simulink model "torque_catalogue"  (R2023b)
settings: Solver=VariableStepAuto  StartTime=0.0  StopTime=10.0  RelTol=1e-3
values from neighbouring files (symbols this model uses):
  ni = 13    [ParameterizeMotorTorqueData.mat]
  nx = 46    [ParameterizeMotorTorqueData.mat]
libraries: fl_lib x20, nesl_utility x9, ee_lib x3
settings Model: Creator=simon  LastModifiedBy=simon
settings SimscapeCC: SimscapeLogType=all  SimscapeLogSimulationStatistics=on

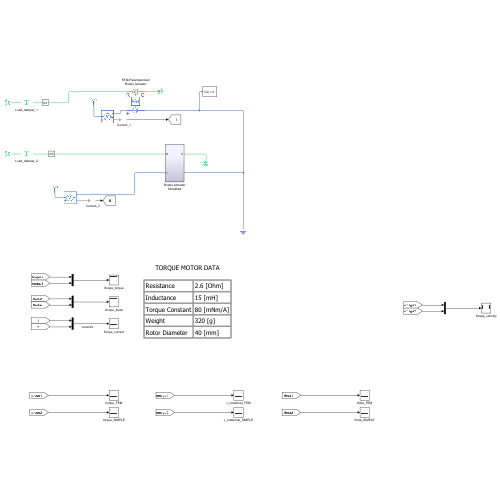
[thumbnail: Simulink's stored preview of the top-level diagram]
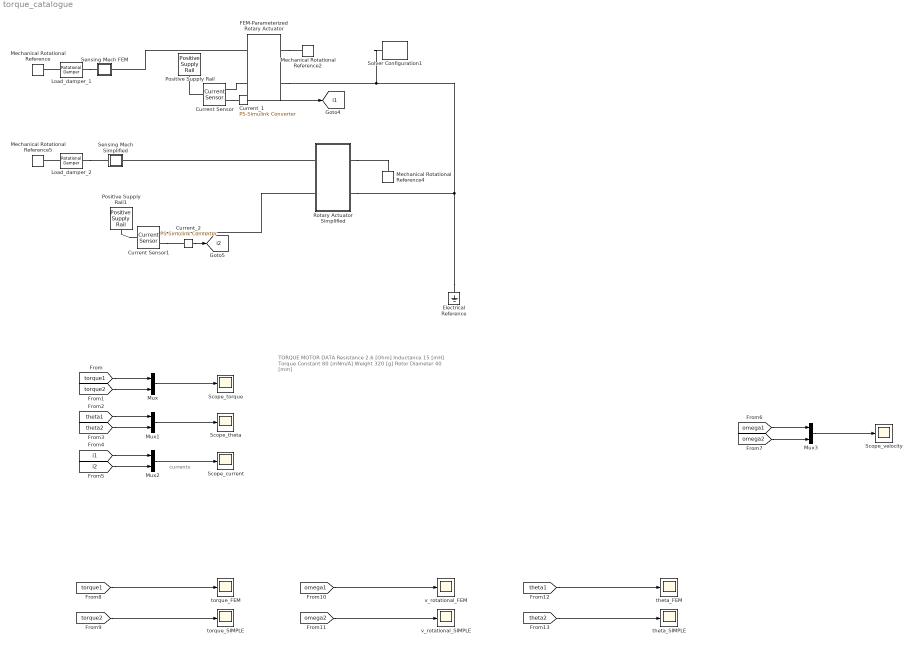
== system torque_catalogue ==
  note: currents
  note: TORQUE MOTOR DATA
      |
      | Resistance
      | 2.6 [Ohm]
      |
      | Inductance
      | 15 [mH]
      |
      | Torque Constant
      | 80 [mNm/A]
      |
      | Weight
      | 320 [g]
      |
      | Rotor Diameter
      | 40 [mm]
  Current Sensor : fl_lib/Electrical/Electrical Sensors/Current Sensor
  Current Sensor1 : fl_lib/Electrical/Electrical Sensors/Current Sensor
  Current_1 : nesl_utility/PS-Simulink Converter  PhysicalDomain=network_engine_domain  SubClassName=ps_output  LeftPortType=input  RightPortType=output  PseudoPeriodic=off  Frequencies=[]  VectorFormat=1-D array  Unit=A  AffineConversion=off
  Current_2 : nesl_utility/PS-Simulink Converter  PhysicalDomain=network_engine_domain  SubClassName=ps_output  LeftPortType=input  RightPortType=output  PseudoPeriodic=off  Frequencies=[]  VectorFormat=1-D array  Unit=A  AffineConversion=off
  Electrical Reference : fl_lib/Electrical/Electrical Elements/Electrical Reference
  FEM-Parameterized Rotary Actuator : ee_lib/Electromechanical/Mechatronic Actuators/FEM-Parameterized Rotary Actuator  src_type=ee.enum.electromech.femRotaryActuator.sourceType.current  iVec=current A  xVec=x rad  dfluxdiMatrix=15e-3*ones(ni,nx) Wb/A  dfluxdxMatrix=dfluxdx Wb/rad  FluxMatrix=[0, 0, 0, 0, 0, 0, 0, 0, 0, 0, 0, 0, 0, 0, 0, 0, 0, 0, 0; .0004, .00048, .0007, .00105, .00147, .00193, .00235, .0027, .00292, .003, .00292, .0027, .00235, .00193, .00147, .00105, .0007, .00048, .0004; .0008, .00096, .00141, .0021, .00295, .00385, .0047, .00539, .00584, .006, .00584, .00539, .0047, .00385, .00295, .0021, .00141, .00096, .0008; .0012, .00144, .00211, .00315, .00442, .00578, .00705, .00809, .00876, .009, .00876, .00809, .00705, .00578, .00442, .00315, .00211, .00144, .0012; .0016, .00191, .00282, .0042, .0059, .0077, .0094, .01078, .01169, .012, .01169, .01078, .0094, .0077, .0059, .0042, .00282, .00191, .0016; .002, .00239, .00352, .00525, .00737, .00963, .01175, .01348, .01461, .015, .01461, .01348, .01175, .00963, .00737, .00525, .00352, .00239, .002] Wb  calculate_torque_matrix=ee.enum.enable.no  TorqueMatrix=torque N*m  cyclic=ee.enum.isCyclic.unique  interp_method=simscape.enum.interpolation.linear  extrap_method=simscape.enum.extrapolation.linear  R1=5.1 Ohm  Rm=inf Ohm  lam=0 N*m*s/rad  Inertia=0.0016 kg*m^2  Xmin=xmin deg  Xmax=xmax deg  K_endstop=1e7 N*m/rad  D_endstop=100 N*m*s/rad  i_specify=off  i_priority=None  i=0 A  i_nominal_specify=off  i_nominal_unit=A  i_nominal_value=1  Trq_specify=off  Trq_priority=None  Trq=0 N*m  Trq_nominal_specify=off  Trq_nominal_unit=N*m  Trq_nominal_value=1  x_specify=on  x_priority=High  x=x0 deg  x_nominal_specify=off  x_nominal_unit=deg  x_nominal_value=1  w_specify=on  w_priority=High  w=0 deg/s  w_nominal_specify=off  w_nominal_unit=deg/s  w_nominal_value=1  magnetic_torque_specify=off  magnetic_torque_priority=None  magnetic_torque=0 N*m  magnetic_torque_nominal_specify=off  magnetic_torque_nominal_unit=N*m  magnetic_torque_nominal_value=1  alpha=3.93e-3 1/K  Tmeas=25 degC  thermal_mass=100 J/K  T_specify=off  T_priority=High  T=300 K  T_nominal_specify=off  T_nominal_unit=K  T_nominal_value=1
      settings: InternalSimscapePortConfiguration="{\"Bottom\":[],\"Left\":[{\"id\":\"p\",\"label\":\"+\",\"type\":\"foundation.electrical.electrical\"},{\"id\":\"R\",\"label\":\"R\",\"type\":\"foundation.mechanical.rotational.rotational\"}],\"Right\":[{\"id\":\"n\",\"label\":\"-\",\"type\":\"foundation.electrical.electrical\"},{\"id\":\"C\",\"label\":\"C\",\"type\":\"foundation.mechanical.rotational.rotational\"}],\"Top\":[]}"
  Load_damper_1 : fl_lib/Mechanical/Rotational Elements/Rotational Damper  D=1 N*m*s/rad  w_specify=off  w_priority=None  w=0 rad/s  w_nominal_specify=off  w_nominal_unit=rad/s  w_nominal_value=1  t_specify=off  t_priority=None  t=0 N*m  t_nominal_specify=off  t_nominal_unit=N*m  t_nominal_value=1
  Load_damper_2 : fl_lib/Mechanical/Rotational Elements/Rotational Damper  D=1 N*m*s/rad  w_specify=off  w_priority=None  w=0 rad/s  w_nominal_specify=off  w_nominal_unit=rad/s  w_nominal_value=1  t_specify=off  t_priority=None  t=0 N*m  t_nominal_specify=off  t_nominal_unit=N*m  t_nominal_value=1
  Mechanical Rotational Reference{,2,4..5} (4 alike) : fl_lib/Mechanical/Rotational Elements/Mechanical Rotational Reference
  Mux{,1..3} (4 alike) : Mux  Inputs=2
  Positive Supply Rail : ee_lib/Sources/Positive Supply Rail  v0=3.5 V
      settings: InternalSimscapePortConfiguration="{\"Bottom\":[],\"Left\":[],\"Right\":[{\"id\":\"p\",\"label\":\"\",\"type\":\"foundation.electrical.electrical\"}],\"Top\":[]}"
  Positive Supply Rail1 : ee_lib/Sources/Positive Supply Rail  v0=3.5 V
      settings: InternalSimscapePortConfiguration="{\"Bottom\":[],\"Left\":[],\"Right\":[{\"id\":\"p\",\"label\":\"\",\"type\":\"foundation.electrical.electrical\"}],\"Top\":[]}"
  "Rotary Actuator Simplified " : Subsystem  Tag=PublishSubsystem
  Scope_current : Scope
  Scope_theta : Scope
  Scope_torque : Scope
  Scope_velocity : Scope
  "Sensing Mech FEM " : Subsystem
      mask Display: disp('m1')
  Sensing Mech Simplified : Subsystem
      mask Display: disp('m2')
  Solver Configuration1 : nesl_utility/Solver Configuration  PhysicalDomain=network_engine_domain  SubClassName=solver  LeftPortType=input  RightPortType=generic  Tones=[]  Harmonics=[]  SimulateNoise=off  Profile=off  UseLocalSampling=off  EnableSwitchedLinearOptims=on  FrequencyDomain=off  UseCCode=off  RelTol=0.001  AbsTol=0.001  MinStep=1e-09  ToWorkspace=off  RevertToSquareIcSolve=off  NumHomotopyIterations=100  PhasorMode=off  PhasorModeNumHarmonics=1  ConsistencySolver=NEWTON_XTOL_AFTER_FTOL  IndexReductionMethod=DerivativeReplacement  DoDC=off  ResidualTolerance=1e-09  ConsistencyTolSource=GLOBAL  ConsistencyAbsTol=0.001  ConsistencyRelTol=0.001  ConsistencyTolFactor=1e-9  UseLocalSolver=off  LocalSolverChoice=NE_BACKWARD_EULER_ADVANCER  ResolveIndetEquations=on  FunctionEvalNumThread=1  LocalSolverSampleTime=0.001  DoFixedCost=off  MaxNonlinIter=3  MaxModeIter=2  ComputeImpulses=off  ImpulseIterations=2  LinearAlgebra=auto  LinearAlgebraNumThread=0  EquationFormulation=NE_TIME_EF  DelaysMemoryBudget=1024  AutomaticFiltering=on  FilteringTimeConstant=0.001  PartitionStorageMethod=AS_NEEDED  PartitionMemoryBudget=1024  PartitionMethod=ROBUST  MultibodyUseLocalSolver=off  MultibodyLocalSolverChoice=ODE1  MultibodyLocalSolverSampleTime=0.001
  theta_FEM : Scope
  theta_SIMPLE : Scope
  torque_FEM : Scope
  torque_SIMPLE : Scope
  v_rotational_FEM : Scope
  v_rotational_SIMPLE : Scope
  tag scope: i1=global, i2=global
  wires:
  [theta2] -> Mux1/2
  [omega1] -> v_rotational_FEM/1
  [theta2] -> theta_SIMPLE/1
  [theta1] -> Mux1/1
  [i1] -> Mux2/1
  Current_1/1 -> [i1]
  [torque2] -> torque_SIMPLE/1
  [torque1] -> Mux/1
  [theta1] -> theta_FEM/1
  [torque1] -> torque_FEM/1
  Mux2/1 -> Scope_current/1
  [omega2] -> Mux3/2
  Mux3/1 -> Scope_velocity/1
  Mux/1 -> Scope_torque/1
  [omega2] -> v_rotational_SIMPLE/1
  [i2] -> Mux2/2
  [torque2] -> Mux/2
  Current_2/1 -> [i2]
  [omega1] -> Mux3/1
  Mux1/1 -> Scope_theta/1
  connections:
  Electrical Reference/LConn1 -- "Rotary Actuator Simplified "/RConn2 -- Solver Configuration1/RConn1 -- FEM-Parameterized Rotary Actuator/RConn1
  Load_damper_2/RConn1 -- Mechanical Rotational Reference5/LConn1
  FEM-Parameterized Rotary Actuator/LConn2 -- "Sensing Mech FEM "/LConn1
  Load_damper_1/RConn1 -- Mechanical Rotational Reference/LConn1
  "Rotary Actuator Simplified "/LConn1 -- Sensing Mech Simplified/LConn1
  Current_1/LConn1 -- Current Sensor/RConn1
  "Rotary Actuator Simplified "/RConn1 -- Mechanical Rotational Reference4/LConn1
  "Rotary Actuator Simplified "/LConn2 -- Current Sensor1/RConn2
  FEM-Parameterized Rotary Actuator/LConn1 -- Current Sensor/RConn2
  Load_damper_2/LConn1 -- Sensing Mech Simplified/RConn1
  Current Sensor1/LConn1 -- Positive Supply Rail1/RConn1
  FEM-Parameterized Rotary Actuator/RConn2 -- Mechanical Rotational Reference2/LConn1
  Load_damper_1/LConn1 -- "Sensing Mech FEM "/RConn1
  Current Sensor1/RConn1 -- Current_2/LConn1
  Current Sensor/LConn1 -- Positive Supply Rail/RConn1

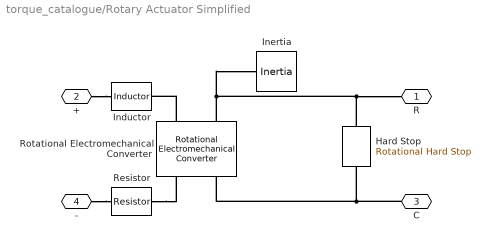
== system torque_catalogue/Rotary Actuator Simplified  ==
  Hard Stop : fl_lib/Mechanical/Rotational Elements/Rotational Hard Stop  upper_bnd=xmax deg  lower_bnd=xmin deg  model=3  stiff_up=1e+7 N*m/rad  stiff_low=1e+7 N*m/rad  D_up=100 N*m/(rad/s)  D_low=100 N*m/(rad/s)  transition=0.001 rad  coeff_rest=0.7  w_tol=0.1 rad/s  trq_tol=0.001 N*m  w_specify=off  w_priority=High  w=0 rad/s  w_nominal_specify=off  w_nominal_unit=rad/s  w_nominal_value=1  t_specify=off  t_priority=High  t=0 N*m  t_nominal_specify=off  t_nominal_unit=N*m  t_nominal_value=1  phi_specify=on  phi_priority=High  phi=x0 deg  phi_nominal_specify=off  phi_nominal_unit=rad  phi_nominal_value=1  M_specify=off  M_priority=None  M=0
  Inductor : fl_lib/Electrical/Electrical Elements/Inductor  l=15 mH  r=0 Ohm  g=1e-9 1/Ohm  i_specify=off  i_priority=High  i=0 A  i_nominal_specify=off  i_nominal_unit=A  i_nominal_value=1  v_specify=off  v_priority=High  v=0 V  v_nominal_specify=off  v_nominal_unit=V  v_nominal_value=1  i_L_specify=on  i_L_priority=High  i_L=0 A  i_L_nominal_specify=off  i_L_nominal_unit=A  i_L_nominal_value=1
  Inertia : fl_lib/Mechanical/Rotational Elements/Inertia  inertia=200 g*cm^2  num_ports=foundation.enum.numPorts2.one  w_specify=on  w_priority=High  w=0 rad/s  w_nominal_specify=off  w_nominal_unit=rad/s  w_nominal_value=1  t_specify=off  t_priority=High  t=0 N*m  t_nominal_specify=off  t_nominal_unit=N*m  t_nominal_value=1
  Resistor : fl_lib/Electrical/Electrical Elements/Resistor  R=2.6 Ohm  i_specify=off  i_priority=High  i=0 A  i_nominal_specify=off  i_nominal_unit=A  i_nominal_value=1  v_specify=off  v_priority=High  v=0 V  v_nominal_specify=off  v_nominal_unit=V  v_nominal_value=1
  Rotational Electromechanical Converter : fl_lib/Electrical/Electrical Elements/Rotational Electromechanical Converter  K=80e-3 V/(rad/s)  i_specify=off  i_priority=High  i=0 A  i_nominal_specify=off  i_nominal_unit=A  i_nominal_value=1  v_specify=off  v_priority=High  v=0 V  v_nominal_specify=off  v_nominal_unit=V  v_nominal_value=1  t_specify=off  t_priority=High  t=0 N*m  t_nominal_specify=off  t_nominal_unit=N*m  t_nominal_value=1  w_specify=off  w_priority=High  w=0 rad/s  w_nominal_specify=off  w_nominal_unit=rad/s  w_nominal_value=1
  R : PMIOPort  Side=Left
  + : PMIOPort  Port=2  Side=Left
  C : PMIOPort  Port=3  Side=Right
  - : PMIOPort  Port=4  Side=Right
  connections:
  +/RConn1 -- Inductor/LConn1
  C/RConn1 -- Rotational Electromechanical Converter/RConn2 -- Hard Stop/RConn1
  -/RConn1 -- Resistor/LConn1
  Resistor/RConn1 -- Rotational Electromechanical Converter/RConn1
  Rotational Electromechanical Converter/LConn1 -- Inductor/RConn1
  Hard Stop/LConn1 -- R/RConn1 -- Rotational Electromechanical Converter/LConn2 -- Inertia/LConn1

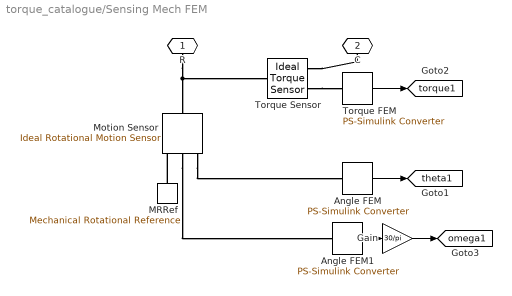
== system torque_catalogue/Sensing Mech FEM  ==
  Angle FEM : nesl_utility/PS-Simulink Converter  PhysicalDomain=network_engine_domain  SubClassName=ps_output  LeftPortType=input  RightPortType=output  PseudoPeriodic=off  Frequencies=[]  VectorFormat=1-D array  Unit=deg  AffineConversion=off
  Angle FEM1 : nesl_utility/PS-Simulink Converter  PhysicalDomain=network_engine_domain  SubClassName=ps_output  LeftPortType=input  RightPortType=output  PseudoPeriodic=off  Frequencies=[]  VectorFormat=1-D array  Unit=rad/s  AffineConversion=off
  Gain : Gain  Gain=30/pi
  MRRef : fl_lib/Mechanical/Rotational Elements/Mechanical Rotational Reference
  Motion Sensor : fl_lib/Mechanical/Mechanical Sensors/Ideal Rotational Motion Sensor  reference=foundation.enum.MeasurementReference.difference  acceleration_port=false  velocity_port=true  position_port=true  wrap_angle=simscape.enum.onoff.off  offset=x0 deg
  Torque FEM : nesl_utility/PS-Simulink Converter  PhysicalDomain=network_engine_domain  SubClassName=ps_output  LeftPortType=input  RightPortType=output  PseudoPeriodic=off  Frequencies=[]  VectorFormat=1-D array  Unit=N*m  AffineConversion=off
  Torque Sensor : fl_lib/Mechanical/Mechanical Sensors/Ideal Torque Sensor
  R : PMIOPort  Side=Left
  C : PMIOPort  Port=2  Side=Right
  tag scope: omega1=global, theta1=global, torque1=global
  wires:
  Angle FEM/1 -> [theta1]
  Torque FEM/1 -> [torque1]
  Angle FEM1/1 -> Gain/1
  Gain/1 -> [omega1]
  connections:
  Torque Sensor/RConn2 -- Torque FEM/LConn1
  Motion Sensor/RConn3 -- Angle FEM/LConn1
  Torque Sensor/RConn1 -- C/RConn1
  R/RConn1 -- Torque Sensor/LConn1 -- Motion Sensor/LConn1
  MRRef/LConn1 -- Motion Sensor/RConn1
  Motion Sensor/RConn2 -- Angle FEM1/LConn1

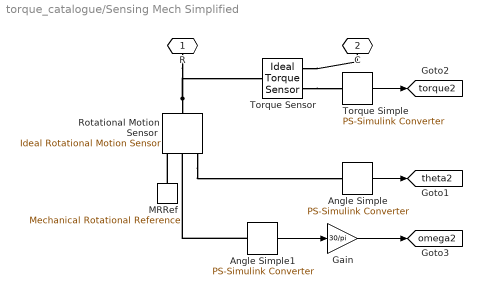
== system torque_catalogue/Sensing Mech Simplified ==
  Angle Simple : nesl_utility/PS-Simulink Converter  PhysicalDomain=network_engine_domain  SubClassName=ps_output  LeftPortType=input  RightPortType=output  PseudoPeriodic=off  Frequencies=[]  VectorFormat=1-D array  Unit=deg  AffineConversion=off
  Angle Simple1 : nesl_utility/PS-Simulink Converter  PhysicalDomain=network_engine_domain  SubClassName=ps_output  LeftPortType=input  RightPortType=output  PseudoPeriodic=off  Frequencies=[]  VectorFormat=1-D array  Unit=rad/s  AffineConversion=off
  Gain : Gain  Gain=30/pi
  MRRef : fl_lib/Mechanical/Rotational Elements/Mechanical Rotational Reference
  Rotational Motion Sensor : fl_lib/Mechanical/Mechanical Sensors/Ideal Rotational Motion Sensor  reference=foundation.enum.MeasurementReference.difference  acceleration_port=false  velocity_port=true  position_port=true  wrap_angle=simscape.enum.onoff.off  offset=x0 deg
  Torque Sensor : fl_lib/Mechanical/Mechanical Sensors/Ideal Torque Sensor
  Torque Simple : nesl_utility/PS-Simulink Converter  PhysicalDomain=network_engine_domain  SubClassName=ps_output  LeftPortType=input  RightPortType=output  PseudoPeriodic=off  Frequencies=[]  VectorFormat=1-D array  Unit=N*m  AffineConversion=off
  R : PMIOPort  Side=Left
  C : PMIOPort  Port=2  Side=Right
  tag scope: omega2=global, theta2=global, torque2=global
  wires:
  Torque Simple/1 -> [torque2]
  Angle Simple/1 -> [theta2]
  Angle Simple1/1 -> Gain/1
  Gain/1 -> [omega2]
  connections:
  MRRef/LConn1 -- Rotational Motion Sensor/RConn1
  Rotational Motion Sensor/LConn1 -- Torque Sensor/LConn1 -- R/RConn1
  Torque Sensor/RConn1 -- C/RConn1
  Rotational Motion Sensor/RConn3 -- Angle Simple/LConn1
  Torque Sensor/RConn2 -- Torque Simple/LConn1
  Angle Simple1/LConn1 -- Rotational Motion Sensor/RConn2
